simulink model "simulink_sim_V1"  (R2023a)
settings: Solver=FixedStepDiscrete  StartTime=0  StopTime=inf  FixedStep=0.001  RelTol=1e-3  EnableMultiTasking=on
values from neighbouring files (symbols this model uses):
  D = zeros(4,2)    [setup_lin_sys.m]
undefined symbols (not defined in the file or in its folder): data, init, pl, sim
libraries: simulink x2
settings Model: Creator=hirsch  LastModifiedBy=srivats
settings SolverCC: AlgebraicLoopSolver=TrustRegion
settings DataIOCC: LimitDataPoints=on  SaveFormat=Array  SignalLoggingSaveFormat=ModelDataLogs  ReturnWorkspaceOutputs=off
settings OptimizationCC: ExpressionDepthLimit=2147483647  LifeSpan=inf
settings DebuggingCC: SolverPrmCheckMsg=warning  FcnCallInpInsideContextMsg=warning  UnconnectedInputMsg=warning  UnconnectedOutputMsg=warning  UnconnectedLineMsg=warning  StateNameClashWarn=warning  SFUnexpectedBacktrackingDiag=warning  SFNoUnconditionalDefaultTransitionDiag=warning  SFExecutionAtInitializationDiag=none  ArithmeticOperatorsInVariantConditions=warning
settings HardwareCC: ProdBitPerPointer=32  ProdBitPerSizeT=32  ProdBitPerPtrDiffT=32  ProdLargestAtomicFloat=None  ProdIntDivRoundTo=Undefined  ProdEndianess=Unspecified  ProdWordSize=32  ProdHWDeviceType=32-bit Generic
settings ModelReferenceCC: EnableRefExpFcnMdlSchedulingChecks=on  PropagateSignalLabelsOutOfModel=off
settings SFSimCC: SimUseLocalCustomCode=off  CustomCodeUndefinedFunction=UseInterfaceOnly
settings RTWCC: RTWUseLocalCustomCode=off
settings CodeAppCC: StateflowObjectComments=on
settings GRTTargetCC: TargetLangStandard=C89/C90 (ANSI)  CombineOutputUpdateFcns=off  GRTInterface=on
settings ConfigComp: CovMetricSettings=dw  CovSaveCumulativeToWorkspaceVar=on  CovSaveSingleToWorkspaceVar=on  CovExternalEMLEnable=off  CovSFcnEnable=off

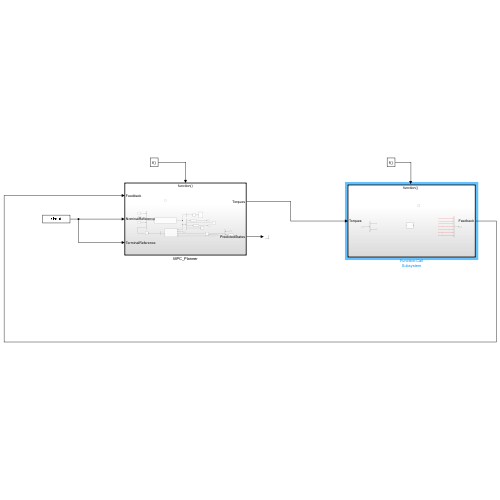
[thumbnail: Simulink's stored preview of the top-level diagram]
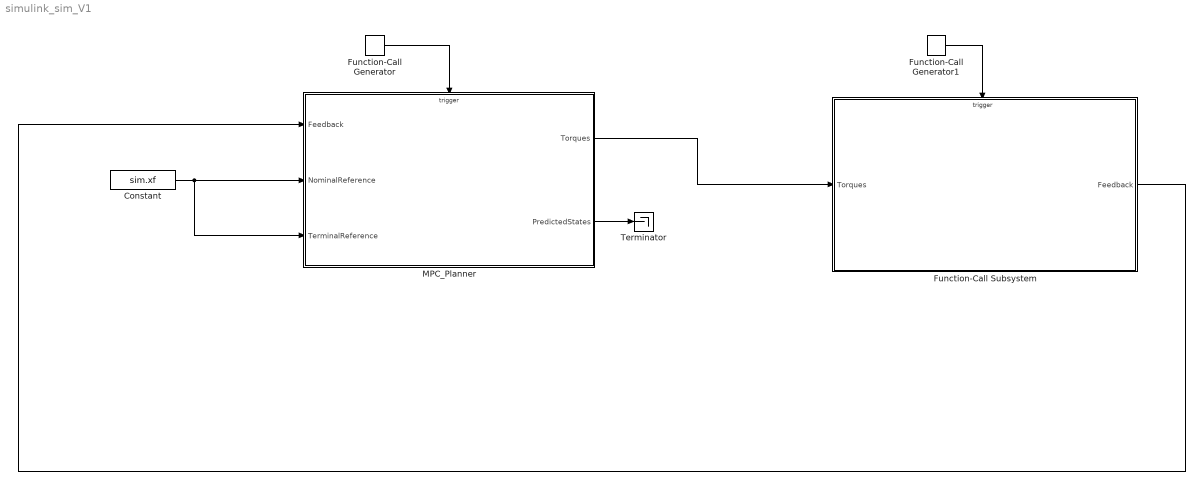
== system simulink_sim_V1 ==
  Constant : Constant  Value=sim.xf
  Function-Call Generator : simulink/Ports & Subsystems/Function-Call Generator  sample_time=pl.Ts  numberOfIterations=1  DisallowWideOutput=off
  Function-Call Generator1 : simulink/Ports & Subsystems/Function-Call Generator  sample_time=0.001  numberOfIterations=1  DisallowWideOutput=off
  Function-Call Subsystem : Subsystem  TreatAsAtomicUnit=on
  MPC_Planner : Subsystem
  Terminator : Terminator
  wires:
  Function-Call Generator/1 -> MPC_Planner/Trigger
  Function-Call Generator1/1 -> Function-Call Subsystem/Trigger
  Function-Call Subsystem/1(Feedback) -> MPC_Planner/1(Feedback)
  MPC_Planner/1(Torques) -> Function-Call Subsystem/1(Torques)
  MPC_Planner/2(PredictedStates) -> Terminator/1
  Constant/1 -> MPC_Planner/3(TerminalReference), MPC_Planner/2(NominalReference)

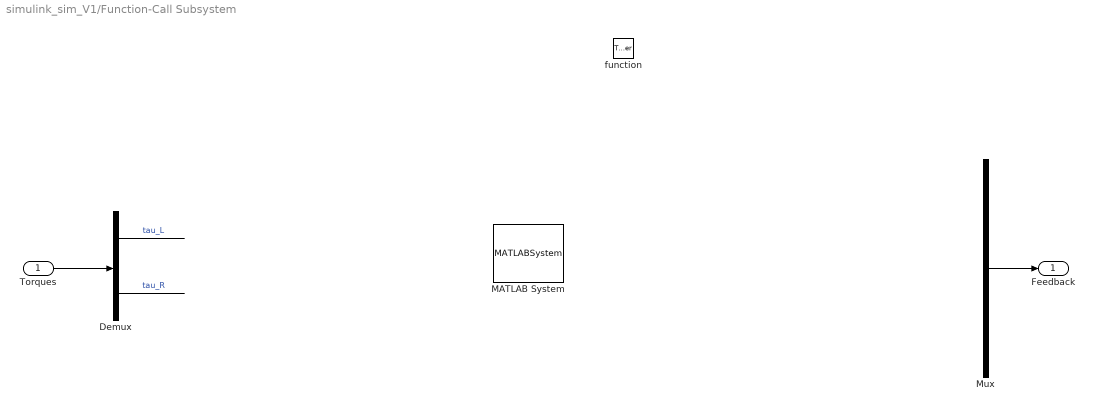
== system simulink_sim_V1/Function-Call Subsystem ==
  Torques : Inport
  function : TriggerPort  TriggerType=function-call  VariantControl=(inherit)
  Demux : Demux  Outputs=2
  MATLAB System : MATLABSystem
  Mux : Mux  Inputs=7
  Feedback : Outport
  wires:
  Torques/1 -> Demux/1
  Demux/1 -> ?  "tau_L"
  Demux/2 -> ?  "tau_R"
  Mux/1 -> Feedback/1
  ? -> Mux/1  "X"
  ? -> Mux/2  "Y"
  ? -> Mux/3  "psi"
  ? -> Mux/4  "v_L"
  ? -> Mux/5  "v_R"
  ? -> Mux/6  "theta"
  ? -> Mux/7  "thetaDot"

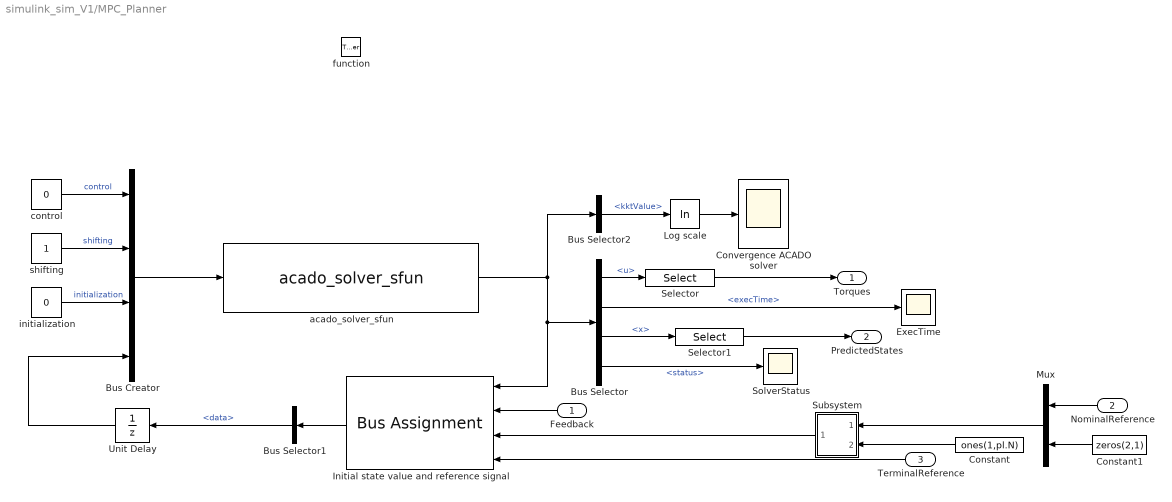
== system simulink_sim_V1/MPC_Planner ==
  Feedback : Inport
  NominalReference : Inport  Port=2
  TerminalReference : Inport  Port=3
  function : TriggerPort  TriggerType=function-call  VariantControl=(inherit)
  Bus Creator : BusCreator  Inputs=4  OutDataTypeStr=Bus: ACADOinput
  Bus Selector : BusSelector  OutputSignals=data.u,execTime,data.x,status
  Bus Selector1 : BusSelector  OutputSignals=data
  Bus Selector2 : BusSelector  OutputSignals=kktValue
  Constant : Constant  Value=ones(1,pl.N)
  Constant1 : Constant  Value=zeros(2,1)
  Convergence ACADO solver : Scope
  ExecTime : Scope
  Initial state value and reference signal : BusAssignment  AssignedSignals=data.x0,data.y,data.yN
  Log scale : Math  Operator=log  SignedPower=on
  Mux : Mux  Inputs=2
  Selector : Selector  InputPortWidth=pl.N  IndexOptions=Starting index (dialog)  Indices=1  OutputSizes=2
  Selector1 : Selector  InputPortWidth=(pl.N+1)*7  IndexOptions=Starting index (dialog)  Indices=1  OutputSizes=7  RuntimeRangeChecks=on
  SolverStatus : Scope
  Subsystem : Subsystem
  Unit Delay : UnitDelay  InitialCondition=init  SampleTime=-1  HasFrameUpgradeWarning=on
  acado_solver_sfun : S-Function  FunctionName=acado_solver_sfun  SFunctionDeploymentMode=off  EnableBusSupport=off  mask(Legacy Function){SFunctionSpec=acado_step(ACADOinput u1[1], ACADOoutput y1[1]), ShowSpec=on}
      mask prompts: ShowSpec "Display function specification"
      mask help:
      | This block allows you to call the legacy functions specified by the following Legacy Code Tool definition:
      | def.SFunctionName = 'acado_solver_sfun';
      | def.OutputFcnSpec = 'acado_step(ACADOinput u1[1], ACADOoutput y1[1])';
      | def.StartFcnSpec = 'acado_initialize( void )';
      | def.TerminateFcnSpec = 'acado_cleanup( void )';
      | def.HeaderFiles = {'acado_common.h', 'acado_solver_sfunction.h'};
      | def.SourceFiles = {'acado_solver.c', 'acado_integrator.c', 'acado_auxiliary_functions.c', 'acado_solver_sfunction.c', 'acado_qpoases3_interface.c', 'qpoases3\src\Bounds.c', 'qpoases3\src\Constraints.c', 'qpoases3\src\Indexlist.c', 'qpoases3\src\Matrices.c', 'qpoases3\src\MessageHandling.c', 'qpoases3\src\Options.c', 'qpoases3\src\Flipper.c', 'qpoases3\src\QProblem.c', 'qpoases3\src\QProblemB.c', 'qpoases3\src\Utils.c'};
      mask Help: <p>This block was generated automatically by the Legacy Code Tool. For detailed help on this tool, call<a href="matlab:legacy_code('help')"> legacy_code('help')</a>.</p>
      mask Callback ShowSpec:
      | if strcmp(get_param(gcbh, 'ShowSpec'), 'on')
      |   set_param(gcbh, 'MaskDisplay', sprintf('fprintf(''%s'');', get_param(gcbh, 'SFunctionSpec')));
      | else
      |   set_param(gcbh, 'MaskDisplay', sprintf('fprintf(''%s'');', get_param(gcbh, 'FunctionName')));
      | end
      mask Display: fprintf('acado_step(ACADOinput u1[1], ACADOoutput y1[1])');
  control : Constant  Value=0  OutDataTypeStr=int32
  initialization : Constant  Value=0  OutDataTypeStr=int32
  shifting : Constant  OutDataTypeStr=int32
  Torques : Outport
  PredictedStates : Outport  Port=2
  wires:
  acado_solver_sfun/1 -> Initial state value and reference signal/1, Bus Selector/1, Bus Selector2/1
  Bus Creator/1 -> acado_solver_sfun/1
  Bus Selector2/1 -> Log scale/1  "<kktValue>"
  Log scale/1 -> Convergence ACADO solver/1
  initialization/1 -> Bus Creator/3  "initialization"
  Initial state value and reference signal/1 -> Bus Selector1/1
  Unit Delay/1 -> Bus Creator/4
  Selector/1 -> Torques/1
  shifting/1 -> Bus Creator/2  "shifting"
  control/1 -> Bus Creator/1  "control"
  Bus Selector/1 -> Selector/1  "<u>"
  Bus Selector1/1 -> Unit Delay/1  "<data>"
  TerminalReference/1 -> Initial state value and reference signal/4
  Feedback/1 -> Initial state value and reference signal/2
  Subsystem/1(Out1) -> Initial state value and reference signal/3
  Bus Selector/2 -> ExecTime/1  "<execTime>"
  Bus Selector/3 -> Selector1/1  "<x>"
  Selector1/1 -> PredictedStates/1
  Bus Selector/4 -> SolverStatus/1  "<status>"
  NominalReference/1 -> Mux/1
  Constant/1 -> Subsystem/2(In2)
  Mux/1 -> Subsystem/1(In1)
  Constant1/1 -> Mux/2

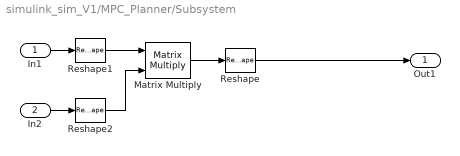
== system simulink_sim_V1/MPC_Planner/Subsystem ==
  In1 : Inport
  In2 : Inport  Port=2
  Matrix Multiply : Product  Multiplication=Matrix(*)
  Reshape : Reshape  OutputDimensionality=Customize  OutputDimensions=[1,pl.N*7+pl.N*2]
  Reshape1 : Reshape  OutputDimensionality=Column vector (2-D)  OutputDimensions=[1,pl.N*7+pl.N*2]
  Reshape2 : Reshape  OutputDimensionality=Row vector (2-D)  OutputDimensions=[1,pl.N*7+pl.N*2]
  Out1 : Outport
  wires:
  Reshape2/1 -> Matrix Multiply/2
  In2/1 -> Reshape2/1
  Reshape1/1 -> Matrix Multiply/1
  Matrix Multiply/1 -> Reshape/1
  In1/1 -> Reshape1/1
  Reshape/1 -> Out1/1
